simulink model "cruise_control_model"  (R2018a)
settings: Solver=ode23t  StartTime=0.0  StopTime=50  RelTol=1e-3
values from neighbouring files (symbols this model uses):
  g = 9.81    [linearized_parameters.m]
  K = 0.07536    [linearized_parameters.m]
  Mv = 1000    [linearized_parameters.m]
  rw = 0.3    [linearized_parameters.m]
undefined symbols (not defined in the file or in its folder): sigbuilder_block
libraries: simulink x2, dspsigops x1
settings Model: Creator=Saurabh Suman  LastModifiedBy=Saurabh Suman

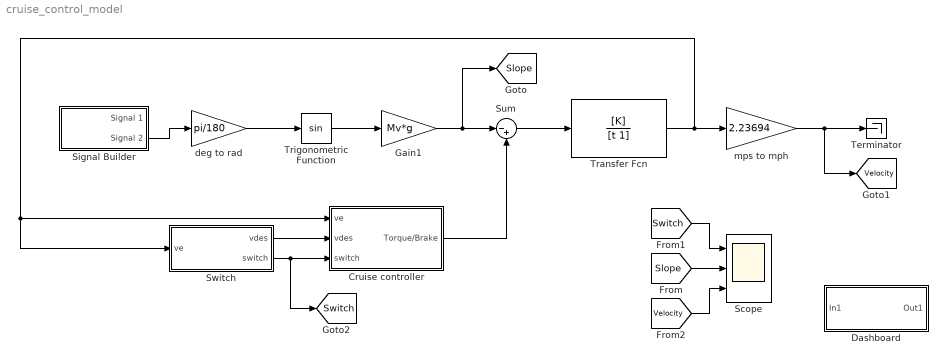
== system cruise_control_model ==
  Cruise controller : Subsystem
  Dashboard : Subsystem
  Gain1 : Gain  Gain=Mv*g
  Scope : Scope  NumInputPorts=3
  Signal Builder : Subsystem  Tag=STV Subsys  LoadFcn=sigbuilder_block('load');  StartFcn=sigbuilder_block('start');  StopFcn=sigbuilder_block('stop');  ClipboardFcn=sigbuilder_block('clipboard');  mask(Sigbuilder block){tuvar=[0:10]}
      mask help: Simulink:masks:SigbuilderBlock_MD
      mask init:
      | if ~strcmp(get_param(bdroot(gcbh),'SimulationStatus'),'stopped') tuvar = sigbuilder_block('maskInit'); end
      settings: CopyFcn=sigbuilder_block('copy');  DeleteFcn=sigbuilder_block('delete');  ModelCloseFcn=sigbuilder_block('modelClose');  PreSaveFcn=sigbuilder_block('preSave');  PauseFcn=sigbuilder_block('pause');  ContinueFcn=sigbuilder_block('continue');  NameChangeFcn=sigbuilder_block('namechange');  OpenFcn=sigbuilder_block('open',[453.6 160.2 550.8 400.2 ]);  CloseFcn=sigbuilder_block('close');
      mask Display: plot(0, 0, 100, 100,[2, 2, 32, 32, 2], [68, 8, 8, 68, 68],[32, 2], [38, 38], [32, 19, 2],[53, 60, 44], [32, 17, 17, 2],[16, 16, 31, 31]);txt = getActiveGroup(gcbh);text(2, 100, txt,'verticalAlignment', 'top');
  Sum : Sum  Inputs=|-+
  Switch : Subsystem
  Terminator : Terminator
  Transfer Fcn : TransferFcn  Numerator=[K]  Denominator=[t 1]
  Trigonometric Function : Trigonometry
  deg to rad : Gain  Gain=pi/180
  mps to mph : Gain  Gain=2.23694
  tag scope: Slope=global, Switch=global, Velocity=global
  wires:
  deg to rad/1 -> Trigonometric Function/1
  Trigonometric Function/1 -> Gain1/1
  Gain1/1 -> [Slope], Sum/1
  Sum/1 -> Transfer Fcn/1
  Transfer Fcn/1 -> Cruise controller/1(ve), Switch/1(ve), mps to mph/1
  mps to mph/1 -> [Velocity], Terminator/1
  Switch/1(vdes) -> Cruise controller/2(vdes)
  Switch/2(switch) -> [Switch], Cruise controller/3(switch)
  Cruise controller/1(Torque/Brake) -> Sum/2
  [Slope] -> Scope/2
  [Velocity] -> Scope/3
  [Switch] -> Scope/1
  Signal Builder/2(Signal 2) -> deg to rad/1

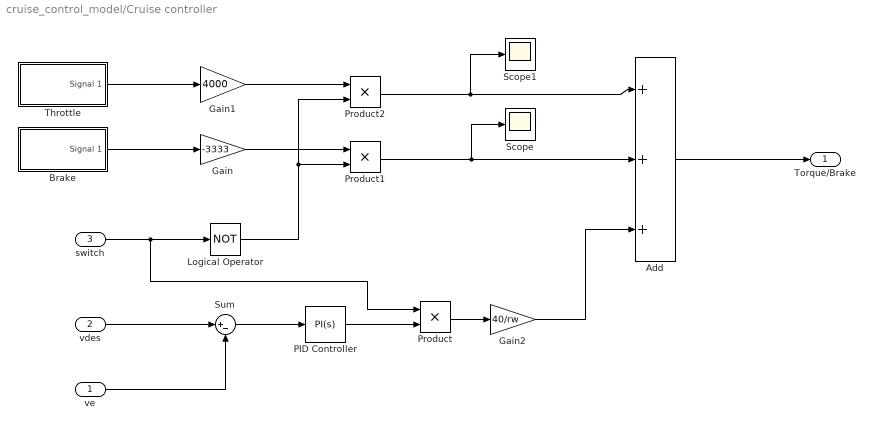
== system cruise_control_model/Cruise controller ==
  ve : Inport
  vdes : Inport  Port=2
  switch : Inport  Port=3
  Add : Sum  Inputs=+++
  Brake : Subsystem  Tag=STV Subsys  LoadFcn=sigbuilder_block('load');  StartFcn=sigbuilder_block('start');  StopFcn=sigbuilder_block('stop');  ClipboardFcn=sigbuilder_block('clipboard');  mask(Sigbuilder block){tuvar=[0:10]}
      mask help: Simulink:masks:SigbuilderBlock_MD
      mask init:
      | if ~strcmp(get_param(bdroot(gcbh),'SimulationStatus'),'stopped') tuvar = sigbuilder_block('maskInit'); end
      settings: CopyFcn=sigbuilder_block('copy');  DeleteFcn=sigbuilder_block('delete');  ModelCloseFcn=sigbuilder_block('modelClose');  PreSaveFcn=sigbuilder_block('preSave');  PauseFcn=sigbuilder_block('pause');  ContinueFcn=sigbuilder_block('continue');  NameChangeFcn=sigbuilder_block('namechange');  OpenFcn=sigbuilder_block('open',[453.6 160.2 550.8 400.2 ]);  CloseFcn=sigbuilder_block('close');
      mask Display: plot(0, 0, 100, 100,[2, 2, 32, 32, 2], [68, 8, 8, 68, 68],[32, 2], [38, 38], [32, 19, 2],[53, 60, 44], [32, 17, 17, 2],[16, 16, 31, 31]);txt = getActiveGroup(gcbh);text(2, 100, txt,'verticalAlignment', 'top');
  Gain : Gain  Gain=-3333
  Gain1 : Gain  Gain=4000
  Gain2 : Gain  Gain=40/rw
  Logical Operator : Logic  Operator=NOT  AllPortsSameDT=off  OutDataTypeStr=boolean
  PID Controller : simulink/Continuous/PID Controller  Controller=PI  TimeDomain=Continuous-time  SampleTime=-1  IntegratorMethod=Forward Euler  FilterMethod=Forward Euler  Form=Parallel  UseFilter=on  ControllerParametersSource=internal  P=10  I=50  D=0  N=100  InitialConditionSource=internal  InitialConditionForIntegrator=0  InitialConditionForFilter=0  ExternalReset=none  LimitOutput=off  UpperSaturationLimit=inf  LowerSaturationLimit=-inf  LinearizeAsGain=on  AntiWindupMode=none  Kb=1  TrackingMode=off  Kt=1  PParamMin=[]  PParamMax=[]  IParamMin=[]  IParamMax=[]  DParamMin=[]  DParamMax=[]  NParamMin=[]  NParamMax=[]  KbParamMin=[]  KbParamMax=[]  KtParamMin=[]  KtParamMax=[]  POutMin=[]  POutMax=[]  IOutMin=[]  IOutMax=[]  DOutMin=[]  DOutMax=[]  NOutMin=[]  NOutMax=[]  KbOutMin=[]  KbOutMax=[]  KtOutMin=[]  KtOutMax=[]  IntegratorOutMin=[]  IntegratorOutMax=[]  FilterOutMin=[]  FilterOutMax=[]  SumOutMin=[]  SumOutMax=[]  SumI1OutMin=[]  SumI1OutMax=[]  SumI2OutMin=[]  SumI2OutMax=[]  SumI3OutMin=[]  SumI3OutMax=[]  SumDOutMin=[]  SumDOutMax=[]  SaturationOutMin=[]  SaturationOutMax=[]  IntegratorContinuousStateAttributes=''  IntegratorStateMustResolveToSignalObject=off  IntegratorRTWStateStorageClass=Auto  FilterContinuousStateAttributes=''  FilterStateMustResolveToSignalObject=off  FilterRTWStateStorageClass=Auto  DifferentiatorICPrevScaledInput=0  DifferentiatorOutMin=[]  DifferentiatorOutMax=[]  FilterDiffOutCoefMin=[]  FilterDiffOutCoefMax=[]  SumDenOutMin=[]  SumDenOutMax=[]  SumNumOutMin=[]  SumNumOutMax=[]  ReciprocalOutMin=[]  ReciprocalOutMax=[]  DivideOutMin=[]  DivideOutMax=[]  TunerSelectOption=Transfer Function Based (PID Tuner App)
  Product : Product
  Product1 : Product
  Product2 : Product
  Scope : Scope
  Scope1 : Scope
  Sum : Sum  Inputs=|+-
  Throttle : Subsystem  Tag=STV Subsys  LoadFcn=sigbuilder_block('load');  StartFcn=sigbuilder_block('start');  StopFcn=sigbuilder_block('stop');  ClipboardFcn=sigbuilder_block('clipboard');  mask(Sigbuilder block){tuvar=[0:10]}
      mask help: Simulink:masks:SigbuilderBlock_MD
      mask init:
      | if ~strcmp(get_param(bdroot(gcbh),'SimulationStatus'),'stopped') tuvar = sigbuilder_block('maskInit'); end
      settings: CopyFcn=sigbuilder_block('copy');  DeleteFcn=sigbuilder_block('delete');  ModelCloseFcn=sigbuilder_block('modelClose');  PreSaveFcn=sigbuilder_block('preSave');  PauseFcn=sigbuilder_block('pause');  ContinueFcn=sigbuilder_block('continue');  NameChangeFcn=sigbuilder_block('namechange');  OpenFcn=sigbuilder_block('open',[453.6 160.2 550.8 400.2 ]);  CloseFcn=sigbuilder_block('close');
      mask Display: plot(0, 0, 100, 100,[2, 2, 32, 32, 2], [68, 8, 8, 68, 68],[32, 2], [38, 38], [32, 19, 2],[53, 60, 44], [32, 17, 17, 2],[16, 16, 31, 31]);txt = getActiveGroup(gcbh);text(2, 100, txt,'verticalAlignment', 'top');
  Torque/Brake : Outport
  wires:
  Throttle/1(Signal 1) -> Gain1/1
  Brake/1(Signal 1) -> Gain/1
  Gain1/1 -> Product2/1
  Gain/1 -> Product1/1
  Logical Operator/1 -> Product1/2, Product2/2
  Product2/1 -> Scope1/1, Add/1
  Product1/1 -> Scope/1, Add/2
  vdes/1 -> Sum/1
  Sum/1 -> PID Controller/1
  PID Controller/1 -> Product/2
  Product/1 -> Gain2/1
  Gain2/1 -> Add/3
  Add/1 -> Torque/Brake/1
  switch/1 -> Product/1, Logical Operator/1
  ve/1 -> Sum/2

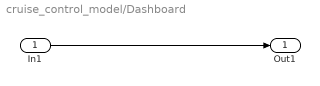
== system cruise_control_model/Dashboard ==
  In1 : Inport
  Out1 : Outport
  wires:
  In1/1 -> Out1/1

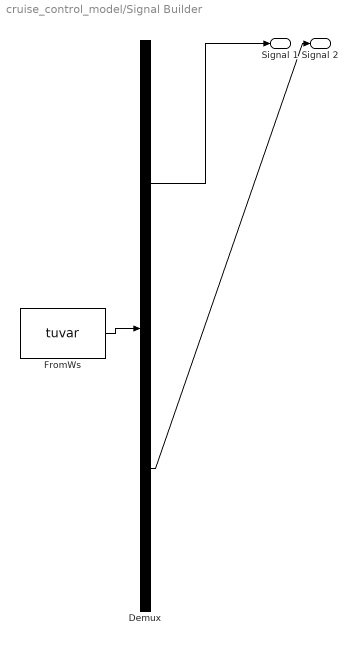
== system cruise_control_model/Signal Builder ==
  Demux : Demux  Tag=STV Demux  Outputs=2
  FromWs : FromWorkspace  Tag=STV FromWs  VariableName=tuvar  SampleTime=0
      SigBuilderData=|
      | common.afterFinalStr = 'Extrapolate'
      | common.sampleTime = 0
      | dataSet(1).timeRange = [0 50]
      | dataSet(1).name = 'Scenario 1'
      | dataSet(2).timeRange = [0 50]
      | dataSet(2).name = 'Scenario 2'
      | sbobj.Groups(1).Name = 'Scenario 1'
      | sbobj.Groups(1).Signals(1).Name = 'Signal 1'
      | sbobj.Groups(1).Signals(1).XData = [0 50]
      | sbobj.Groups(1).Signals(1).YData = [0 0]
      | sbobj.Groups(1).Signals(2).Name = 'Signal 2'
      | sbobj.Groups(1).Signals(2).XData = [0 20 20 30 30 50]
      | sbobj.Groups(1).Signals(2).YData = [0 0 1 1 0 0]
      | sbobj.Groups(1).TimeRange = [0 50]
      | sbobj.Groups(2).Name = 'Scenario 2'
      | sbobj.Groups(2).Signals(1).Name = 'Signal 1'
      | sbobj.Groups(2).Signals(1).XData = [0 15 15 25 25 50]
      | sbobj.Groups(2).Signals(1).YData = [0 0 5 5 0 0]
      | sbobj.Groups(2).Signals(2).Name = 'Signal 2'
      | sbobj.Groups(2).Signals(2).XData = [0 15 15 25 25 50]
      | sbobj.Groups(2).Signals(2).YData = [0 0 -5 -5 0 0]
      | sbobj.Groups(2).TimeRange = [0 50]
  Signal 1 : Outport  Tag=STV Outport
  Signal 2 : Outport  Tag=STV Outport  Port=2
  wires:
  Demux/1 -> Signal 1/1
  FromWs/1 -> Demux/1
  Demux/2 -> Signal 2/1

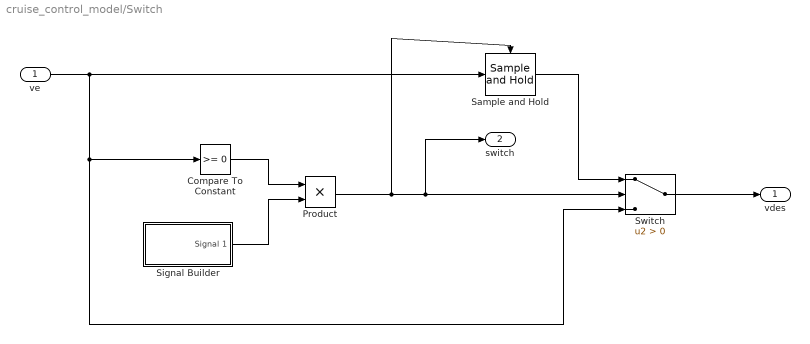
== system cruise_control_model/Switch ==
  ve : Inport
  Compare To Constant : simulink/Logic and Bit Operations/Compare To Constant  relop=>=  const=0  OutDataTypeStr=boolean
  Product : Product
  Sample and Hold : dspsigops/Sample and Hold  trig=Rising edge  initCond=0  latchinput=off
  Signal Builder : Subsystem  Tag=STV Subsys  LoadFcn=sigbuilder_block('load');  StartFcn=sigbuilder_block('start');  StopFcn=sigbuilder_block('stop');  ClipboardFcn=sigbuilder_block('clipboard');  mask(Sigbuilder block){tuvar=[0:10]}
      mask help: Simulink:masks:SigbuilderBlock_MD
      mask init:
      | if ~strcmp(get_param(bdroot(gcbh),'SimulationStatus'),'stopped') tuvar = sigbuilder_block('maskInit'); end
      settings: CopyFcn=sigbuilder_block('copy');  DeleteFcn=sigbuilder_block('delete');  ModelCloseFcn=sigbuilder_block('modelClose');  PreSaveFcn=sigbuilder_block('preSave');  PauseFcn=sigbuilder_block('pause');  ContinueFcn=sigbuilder_block('continue');  NameChangeFcn=sigbuilder_block('namechange');  OpenFcn=sigbuilder_block('open',[453.6 160.2 550.8 400.2 ]);  CloseFcn=sigbuilder_block('close');
      mask Display: plot(0, 0, 100, 100,[2, 2, 32, 32, 2], [68, 8, 8, 68, 68],[32, 2], [38, 38], [32, 19, 2],[53, 60, 44], [32, 17, 17, 2],[16, 16, 31, 31]);txt = getActiveGroup(gcbh);text(2, 100, txt,'verticalAlignment', 'top');
  Switch : Switch  Criteria=u2 > Threshold
  vdes : Outport
  switch : Outport  Port=2
  wires:
  ve/1 -> Compare To Constant/1, Switch/3, Sample and Hold/1
  Compare To Constant/1 -> Product/1
  Signal Builder/1(Signal 1) -> Product/2
  Product/1 -> Sample and Hold/Trigger, switch/1, Switch/2
  Sample and Hold/1 -> Switch/1
  Switch/1 -> vdes/1

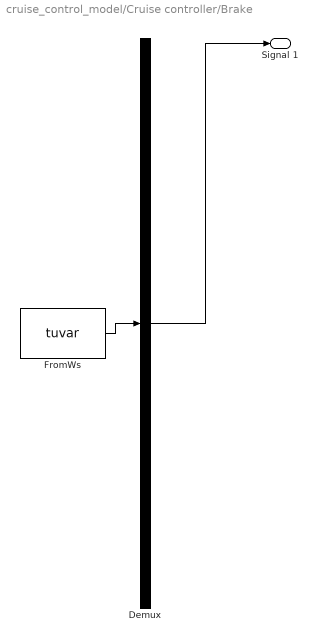
== system cruise_control_model/Cruise controller/Brake ==
  Demux : Demux  Tag=STV Demux  Outputs=1
  FromWs : FromWorkspace  Tag=STV FromWs  VariableName=tuvar  SampleTime=0
      SigBuilderData=|
      | common.afterFinalStr = 'Extrapolate'
      | common.sampleTime = 0
      | dataSet.timeRange = [0 50]
      | dataSet.name = 'Scenario 1&2'
      | sbobj.Groups.Name = 'Scenario 1&2'
      | sbobj.Groups.Signals.Name = 'Signal 1'
      | sbobj.Groups.Signals.XData = [0 45 45 50]
      | sbobj.Groups.Signals.YData = [0 0 0.4 0.4]
      | sbobj.Groups.TimeRange = [0 50]
  Signal 1 : Outport  Tag=STV Outport
  wires:
  Demux/1 -> Signal 1/1
  FromWs/1 -> Demux/1

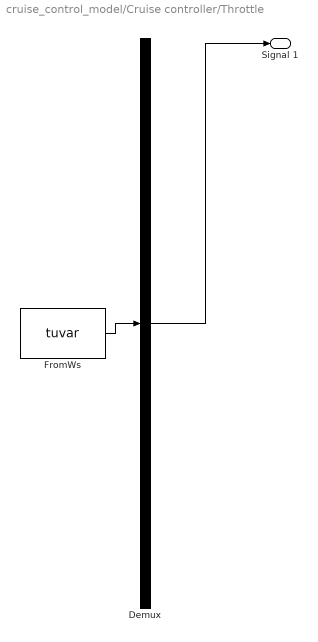
== system cruise_control_model/Cruise controller/Throttle ==
  Demux : Demux  Tag=STV Demux  Outputs=1
  FromWs : FromWorkspace  Tag=STV FromWs  VariableName=tuvar  SampleTime=0
      SigBuilderData=|
      | common.afterFinalStr = 'Extrapolate'
      | common.sampleTime = 0
      | dataSet.timeRange = [0 50]
      | dataSet.name = 'Scenario 1&2'
      | sbobj.Groups.Name = 'Scenario 1&2'
      | sbobj.Groups.Signals.Name = 'Signal 1'
      | sbobj.Groups.Signals.XData = [0 10 10 30 30 40 45 50]
      | sbobj.Groups.Signals.YData = [0.5 0.3 0 0 0.3 0.3 0 0]
      | sbobj.Groups.TimeRange = [0 50]
  Signal 1 : Outport  Tag=STV Outport
  wires:
  Demux/1 -> Signal 1/1
  FromWs/1 -> Demux/1

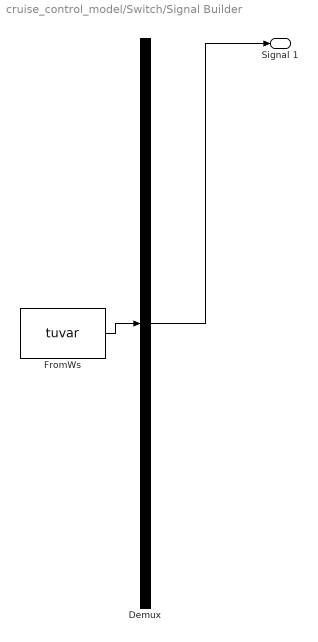
== system cruise_control_model/Switch/Signal Builder ==
  Demux : Demux  Tag=STV Demux  Outputs=1
  FromWs : FromWorkspace  Tag=STV FromWs  VariableName=tuvar  SampleTime=0
      SigBuilderData=|
      | common.afterFinalStr = 'Extrapolate'
      | common.sampleTime = 0
      | dataSet.timeRange = [0 50]
      | dataSet.name = 'Group 1'
      | sbobj.Groups.Name = 'Group 1'
      | sbobj.Groups.Signals.Name = 'Signal 1'
      | sbobj.Groups.Signals.XData = [0 10 10 30 30 50]
      | sbobj.Groups.Signals.YData = [0 0 1 1 0 0]
      | sbobj.Groups.TimeRange = [0 50]
  Signal 1 : Outport  Tag=STV Outport
  wires:
  Demux/1 -> Signal 1/1
  FromWs/1 -> Demux/1
